simulink model "ftbf_old"  (R2018a)
settings: Solver=VariableStepAuto  StartTime=0.0  StopTime=1  RelTol=1e-3
values from neighbouring files (symbols this model uses):
  dC = dC{1}    [Trottinette.m]    (also in Trottinette_2.m; Trottinette_couple.m; Trottinette_vitesse.m)
  dF = dF{1}    [Trottinette.m]    (also in Trottinette_2.m; Trottinette_couple.m; Trottinette_vitesse.m)
  dG = dG{1}    [Trottinette.m]    (also in Trottinette_couple.m)
  E = 0    [Trottinette.m]    (also in Trottinette_couple.m)
  nC = nC{1}    [Trottinette.m]    (also in Trottinette_2.m; Trottinette_couple.m; Trottinette_vitesse.m)
  nF = nF{1}    [Trottinette.m]    (also in Trottinette_2.m; Trottinette_couple.m; Trottinette_vitesse.m)
  nG = nG{1}    [Trottinette.m]    (also in Trottinette_couple.m)
settings Model: Creator=heusse  LastModifiedBy=mluser
settings DataIOCC: ReturnWorkspaceOutputs=on
settings SFSimCC: SimUseLocalCustomCode=on
settings RTWCC: RTWUseLocalCustomCode=on

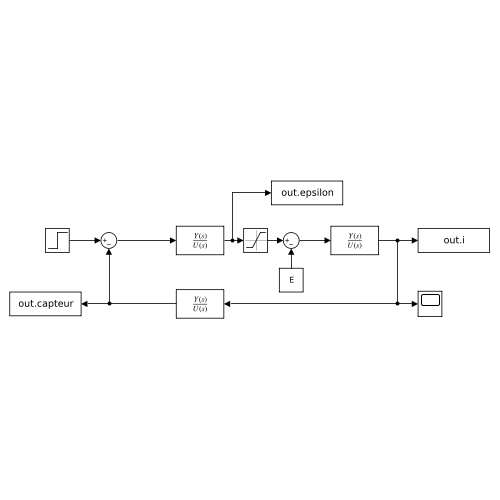
[thumbnail: Simulink's stored preview of the top-level diagram]
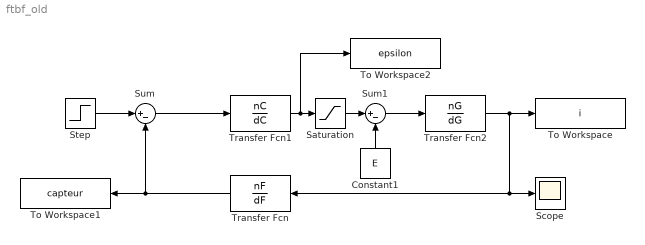
== system ftbf_old ==
  Constant1 : Constant  Value=E
  Saturation : Saturate
  Scope : Scope
  Step : Step  Time=0  After=0.3  SampleTime=0
  Sum : Sum  Inputs=|+-
  Sum1 : Sum  Inputs=|+-
  To Workspace : ToWorkspace  VariableName=i  SaveFormat=Timeseries  SampleTime=-1
  To Workspace1 : ToWorkspace  VariableName=capteur  SaveFormat=Timeseries  SampleTime=-1
  To Workspace2 : ToWorkspace  VariableName=epsilon  SaveFormat=Timeseries  SampleTime=-1
  Transfer Fcn : TransferFcn  Numerator=nF  Denominator=dF
  Transfer Fcn1 : TransferFcn  Numerator=nC  Denominator=dC
  Transfer Fcn2 : TransferFcn  Numerator=nG  Denominator=dG
  wires:
  Step/1 -> Sum/1
  Sum/1 -> Transfer Fcn1/1
  Transfer Fcn/1 -> To Workspace1/1, Sum/2
  Sum1/1 -> Transfer Fcn2/1
  Transfer Fcn1/1 -> To Workspace2/1, Saturation/1
  Transfer Fcn2/1 -> To Workspace/1, Transfer Fcn/1, Scope/1
  Constant1/1 -> Sum1/2
  Saturation/1 -> Sum1/1
